simulink model "PlantaV4_6_prueba_contacto_4"  (R2021a)
settings: Solver=VariableStepAuto  StartTime=0.0  StopTime=60  MaxStep=1e-2  RelTol=1e-3
values from neighbouring files (symbols this model uses):
  ahmax = 0.75    [valoresPlanta_29_9_24.m]    (also in valoresPlanta_V3.m)
  alfahmax = ((2*ahmax)/(rhd))    (= 2)    [valoresPlanta_29_9_24.m]    (also in valoresPlanta_V3.m)
  alfatmax = atmax/rtd    (= 1.6)    [valoresPlanta_29_9_24.m]    (also in valoresPlanta_V3.m)
  atmax = 0.8    [valoresPlanta_29_9_24.m]    (also in valoresPlanta_V3.m)
  ax_max = 0.8    [valoresPlanta_29_9_24.m]    (also in valoresPlanta_v4.m)
  ay_max = 0.75    [valoresPlanta_29_9_24.m]    (also in valoresPlanta_v4.m)
  bcx = 1e6    (= 1000000)    [Valores_1.m]    (also in valoresPlanta.m; valoresPlanta_29_9_24.m; valoresPlanta_V3.m; valoresPlanta_v4.m)
  bcy = 1e7    (= 10000000)    [Valores_1.m]    (also in valoresPlanta.m; valoresPlanta_29_9_24.m; valoresPlanta_V3.m; valoresPlanta_v4.m)
  bh_eq = bhm*ih^2+bhd    (= 8720)    [Valores.m]    (also in Valores_1.m; valoresPlanta.m; valoresPlanta_29_9_24.m; valoresPlanta_V3.m)
  bhb = 1e8    (= 100000000)    [Valores.m]    (also in Valores_1.m; valoresPlanta.m; valoresPlanta_29_9_24.m; valoresPlanta_V3.m)
  bhEb = 2.2e9    (= 2200000000)    [Valores.m]    (also in Valores_1.m; valoresPlanta.m; valoresPlanta_29_9_24.m; valoresPlanta_V3.m)
  bt = 90.0    (= 90)    [Valores.m]    (also in Valores_1.m; valoresPlanta.m; valoresPlanta_29_9_24.m; valoresPlanta_V3.m)
  bt_eq = btd+(btm*(it^2))    (= 5401.8)    [valoresPlanta.m]    (also in valoresPlanta_29_9_24.m; valoresPlanta_V3.m; valoresPlanta_v4.m)
  btw = 3.0e3    (= 3000)    [Valores.m]    (also in Valores_1.m; valoresPlanta.m; valoresPlanta_29_9_24.m; valoresPlanta_V3.m)
  bwu = 150    [Valores.m]    (also in Valores_1.m; valoresPlanta.m; valoresPlanta_29_9_24.m; valoresPlanta_V3.m)
  estado_cont = [x_positions; hy_cont]    [perfilObsaculos.m]    (also in valoresPlanta_29_9_24.m = [x_positions; [hy_muelle hy_cont]])
  g = 9.80665    [Valores.m]    (also in Valores_1.m; valoresPlanta.m; valoresPlanta_29_9_24.m; valoresPlanta_V3.m)
  Hc = 0    [Valores.m]    (also in Valores_1.m = 2.5; valoresPlanta.m = 2.5; valoresPlanta_29_9_24.m = 2.5; valoresPlanta_V3.m = 2.5)
  hMax = 10    [Valores_1.m]    (also in valoresPlanta.m; valoresPlanta_V3.m; valoresPlanta_v4.m)
  hx_cont = 2.5    [perfilObsaculos.m]    (also in puntosTrayectoria.m; valoresPlanta_29_9_24.m)
  ih = 22    [Valores.m]    (also in Valores_1.m; valoresPlanta.m; valoresPlanta_29_9_24.m; valoresPlanta_V3.m)
  it = 30    [Valores.m]    (also in Valores_1.m; valoresPlanta.m; valoresPlanta_29_9_24.m; valoresPlanta_V3.m)
  Jh_eq = Jhm_hb*ih^2+Jhd_hEb    (= 18320)    [Valores.m]    (also in Valores_1.m; valoresPlanta.m; valoresPlanta_29_9_24.m; valoresPlanta_V3.m)
  Jt_eq = Jtd+(Jtm_tb*(it^2))    (= 7500)    [valoresPlanta.m]    (also in valoresPlanta_29_9_24.m; valoresPlanta_V3.m; valoresPlanta_v4.m)
  kcy = 1.8e9    (= 1800000000)    [Valores_1.m]    (also in valoresPlanta.m; valoresPlanta_29_9_24.m; valoresPlanta_V3.m; valoresPlanta_v4.m)
  KDh = Jeq2 * w_posh^3    (= -12245.4404091)    [Valores.m]    (also in Valores_1.m = Jeq2 * w_posh; valoresPlanta.m = Jeq2 * w_posh; valoresPlanta_29_9_24.m = Jh_eq * n * w_posh; valoresPlanta_V3.m = Jeq2 * w_posh)
  KDt = Meq2 * w_post^3    (= -4728.86946035)    [Valores.m]    (also in Valores_1.m = Meq2 * w_post; valoresPlanta.m = Meq2 * w_post; valoresPlanta_29_9_24.m = 10127; valoresPlanta_V3.m = Meq2 * w_post)
  KIh = Jeq2 * w_posh^2    (= 2572.66592082)    [Valores.m]    (also in Valores_1.m = Jeq2 * w_posh^3; valoresPlanta.m = Jeq2 * w_posh^3; valoresPlanta_29_9_24.m = Jh_eq * w_posh^3; valoresPlanta_V3.m = Jeq2 * w_posh^3)
  KIt = Meq2 * w_post^2    (= 1307.690244)    [Valores.m]    (also in Valores_1.m = Meq2 * w_post^3; valoresPlanta.m = Meq2 * w_post^3; valoresPlanta_29_9_24.m = 6809.6; valoresPlanta_V3.m = Meq2 * w_post^3)
  KPh = Jeq2 * w_posh    (= -540.495867769)    [Valores.m]    (also in Valores_1.m = Jeq2 * w_posh^2; valoresPlanta.m = Jeq2 * w_posh^2; valoresPlanta_29_9_24.m = Jh_eq * n * w_posh^2; valoresPlanta_V3.m = Jeq2 * w_posh^2)
  KPt = Meq2 * w_post    (= -361.62)    [Valores.m]    (also in Valores_1.m = Meq2 * w_post^2; valoresPlanta.m = Meq2 * w_post^2; valoresPlanta_29_9_24.m = 14123; valoresPlanta_V3.m = Meq2 * w_post^2)
  Ktw = 4.8e5    (= 480000)    [Valores.m]    (also in Valores_1.m; valoresPlanta.m; valoresPlanta_29_9_24.m; valoresPlanta_V3.m)
  kwu = 2.36e8    (= 236000000)    [Valores.m]    (also in Valores_1.m; valoresPlanta.m; valoresPlanta_29_9_24.m; valoresPlanta_V3.m)
  Mc_max = 5e4    (= 50000)    [Valores.m]    (also in Valores_1.m; valoresPlanta.m; valoresPlanta_29_9_24.m; valoresPlanta_V3.m)
  Mc_min = 2e3    (= 2000)    [Valores.m]    (also in Valores_1.m; valoresPlanta.m; valoresPlanta_29_9_24.m; valoresPlanta_V3.m)
  Meq = Mt+(it^2*Jtm_tb+Jtd)/rtd^2    (= 60000)    [Valores.m]    (also in Valores_1.m; valoresPlanta_29_9_24.m; valoresPlanta_v4.m)
  Ms = 1.5e4    (= 15000)    [Valores.m]    (also in Valores_1.m; valoresPlanta.m; valoresPlanta_29_9_24.m; valoresPlanta_V3.m)
  Mt = 30000    [Valores.m]    (also in Valores_1.m; valoresPlanta.m; valoresPlanta_29_9_24.m; valoresPlanta_V3.m)
  rhd = 0.75    [Valores.m]    (also in Valores_1.m; valoresPlanta.m; valoresPlanta_29_9_24.m; valoresPlanta_V3.m)
  rtd = 0.5    [Valores.m]    (also in Valores_1.m; valoresPlanta.m; valoresPlanta_29_9_24.m; valoresPlanta_V3.m)
  tau_hm = 1e-3    (= 0.001)    [valoresPlanta.m]    (also in valoresPlanta_29_9_24.m; valoresPlanta_V3.m; valoresPlanta_v4.m)
  tau_tm = 1e-3    (= 0.001)    [Valores.m]    (also in Valores_1.m; valoresPlanta.m; valoresPlanta_29_9_24.m; valoresPlanta_V3.m)
  Thb_Max = 5e4    (= 50000)    [Valores.m]    (also in Valores_1.m; valoresPlanta.m; valoresPlanta_29_9_24.m; valoresPlanta_V3.m)
  ThEb_Max = 1.1e6    (= 1100000)    [Valores.m]    (also in Valores_1.m; valoresPlanta.m; valoresPlanta_29_9_24.m; valoresPlanta_V3.m)
  Thm_Max = 2e4    (= 20000)    [Valores.m]    (also in Valores_1.m; valoresPlanta.m; valoresPlanta_29_9_24.m; valoresPlanta_V3.m)
  Ttb_Max = 5e3    (= 5000)    [Valores.m]    (also in Valores_1.m; valoresPlanta.m; valoresPlanta_29_9_24.m; valoresPlanta_V3.m)
  Ttm_Max = 3e3    (= 3000)    [Valores.m]    (also in Valores_1.m; valoresPlanta.m; valoresPlanta_29_9_24.m = 4000; valoresPlanta_V3.m)
  v_x_max = 4    [Valores_1.m]    (also in valoresPlanta.m; valoresPlanta_V3.m = 0.4; valoresPlanta_v4.m)
  vx_max = 4    [valoresPlanta_29_9_24.m]
  y0 = 2.5    [valoresPlanta_29_9_24.m]
  Yt0 = 45    [Valores.m]    (also in Valores_1.m; valoresPlanta.m; valoresPlanta_29_9_24.m; valoresPlanta_V3.m)
undefined symbols (not defined in the file or in its folder): sigbuilder_block, x0
libraries: vrlib x1, simulink_extras x1, cstblocks x1
(part 2 of 2)

== stateflow chart PlantaV4_6_prueba_contacto_4/Control Supervisor/Movimiento ==
  state estado_inicial [parallel] [commented out]
    entry:
    vYref = 0;
    vXref = 0;
    flag_carga = 1;
  state Movimiento [parallel] [commented out]
    entry:
    h_i = 0;
    h_seg = 0;
    %[h_i, h_seg] = calculaH1(v_x_max, dX, hMax, v_y_max,dh);
    %v_x_max = 4;
    during:
    v_y_max = calcVel(ml, g);
    %v_y_max = 2;
    h_i = 5;
    h_seg = 15;
    %[h_i, h_seg] = calculaH1(v_x_max, dX, hMax, v_y_max,dh);
    state Estado4 [commented out]
      entry:
      E = 4; %estado 4
      during:
      if (toDock==1)
      vYref = v_y_max; %suma
      vXref = v_x_max;  %cte desaceleracion hasta 0 (suma)
      else
      vYref = v_y_max; %suma
      vXref = 0.1;  %cte desaceleracion hasta 0
      end
    state Estado3 [commented out]
      entry:
      E = 3; %estado 3
      during:
      vYref = 0;
      if (toDock==1)
      vXref = -v_x_max;
      else
      vXref = v_x_max;
      end
    state Estado2 [commented out]
      entry:
      E = 2; %estado 2
      during:
      if (toDock==1)
      vYref = -v_y_max;
      vXref = -v_x_max;
      else
      vYref = v_y_max;
      vXref = v_x_max;
      end
    note: %ver de comparar con posicion objetivo
        | definir hmax (2 contenedores)
    state DescargaConteiner [commented out]
      entry:
      ml = Ms;
    state Estado5 [commented out]
      entry:
      E = 5; %estado 5
      during:
      if (toDock==1)
      vYref = vYref+0.5; %acelero
      vXref = 0;
      %ml = Ms;
      else
      vYref = vYref-0.5; %desacelero
      vXref = 0;
      end
    state Estado1 [commented out]
      entry:
      E = 1; %estado 1
      during:
      if (toDock==1)
      if (yl > 0)
      vYref = -v_y_max;
      end
      else
      vYref = v_y_max;
      if (yl < h_i)
      vYref = 0;
      end
      end
    state EstadoInicial [commented out]
      entry:
      entry:
      E = 0; %estado 0
      vYref = 0;
      vXref = 0;
      flag_carga = 0;
      ml = fcn(Mc_Max, Mc_Min);
    Estado3 -> Estado2 [commented out] : [xl<=dX && toDock==1 && yl >= h_seg]
    Estado3 -> Estado4 [commented out] : [xl>= posXref-7.5 && toDock==0]
    Estado2 -> Estado3 [commented out] : [xl>=dX && toDock==0 && yl >= h_seg]
    Estado4 -> Estado3 [commented out] : [xl<= posXref-7.5 && toDock==1]
    Estado4 -> Estado5 [commented out] : [yl==hMax && vXref<=0 && toDock==0]
    Estado5 -> Estado4 [commented out] : [yl==hMax && toDock==1]
    Estado2 -> Estado1 [commented out] : [yl<=h_i && toDock==1]
    Estado1 -> Estado2 [commented out] : [yl >= h_i && toDock==0]
    Estado5 -> DescargaConteiner [commented out] : [yl == posYref && toDock==0]
    DescargaConteiner -> EstadoInicial [commented out] : [Automatico == 1 && flag_carga == 1]
    (default) -> EstadoInicial [commented out]
    EstadoInicial -> Estado1 [commented out] : [Automatico == 1 && toDock==0]
    EstadoInicial -> Estado5 [commented out] : [Automatico == 1 && toDock==1]
    Estado1 -> EstadoInicial [commented out] : [Automatico == 1 && toDock==1]
  state Manual [parallel] [commented out]
  state estado_inicial1 [parallel] [commented out]
    entry:
    vYref = 0;
    vXref = 0;
    flag_carga = 1;
  state perfiles [parallel]
    entry:
    v_y_max = calcVel(ml, g);
    v_x_max = vx_max;
    during:
    h_i = pos(1,2);
    h_seg = pos(2,2);
    ds = pos(3,2) - pos(1,2);
    db = pos(4,2) - pos(6,2);
    y2 = ds - calcPos(ds, v_y_max, ahmax,0);
    y3 = db - calcPos(db, v_y_max, ahmax,0);
    %funcionaria para 1 ciclo, sino calcular x2 en carro
    %x2 = 10;
    dc = pos(5,1) - pos(2,1);
    x2 = dc - calcPos(dc, v_x_max, ax_max,0);
    vXref = 0;
    vYref = 0;
    settings: executionOrder=1
    state izaje1 [parallel]
      settings: executionOrder=2
      state inicial
        entry:
      state Izaje_subida
        state trayectoria
          entry:
          initialTime_y = currentTime;  %10
          % perfil de velocidad teniendo en cuenta el tiempo, no el espacio a alcanzar
          % totalTime: tiempo necesario para llegar al x final
          if (estado==1)
          PosFinal_y = pos(3,2)-pos(1,2);
          elseif (estado==6)
          PosFinal_y = pos2(3,2)-pos2(1,2);
          end
          %no se si se puede redefinir asi v_max
          [totalTime_y, v_y_max] = calcularTiempoTrapezoidal(PosFinal_y, v_y_max, ay_max);
          vYref = generateVelocityProfile(v_y_max, ay_max, currentTime, totalTime_y, initialTime_y);
          during:
          vYref = generateVelocityProfile(v_y_max, ay_max, currentTime, totalTime_y, initialTime_y);
        state detencion
          entry:
          vYref = 0;
          during:
          vYref = 0;
        perfiles.izaje1.Izaje_subida.trayectoria -> perfiles.izaje1.Izaje_subida.detencion : [estado==3 || estado == 8]
      state Izaje_bajada
        state trayectoria
          entry:
          initialTime_y = currentTime;  %10
          % perfil de velocidad teniendo en cuenta el tiempo, no el espacio a alcanzar
          % totalTime: tiempo necesario para llegar al x final
          if (estado == 4)
          PosFinal_y = abs(pos(6,2)-pos(4,2));
          elseif (estado == 9)
          PosFinal_y = abs(pos2(6,2)-pos2(4,2));
          end
          [totalTime_y, v_y_max] = calcularTiempoTrapezoidal(PosFinal_y, v_y_max, ay_max);
          vYref = - generateVelocityProfile(v_y_max, ay_max, currentTime, totalTime_y, initialTime_y);
          during:
          vYref = - generateVelocityProfile(v_y_max, ay_max, currentTime, totalTime_y, initialTime_y);
        state detencion
          entry:
          vYref = 0;
          during:
          vYref = 0;
        perfiles.izaje1.Izaje_bajada.trayectoria -> perfiles.izaje1.Izaje_bajada.detencion : [estado==6 || estado==11]
      perfiles.izaje1.inicial -> perfiles.izaje1.Izaje_subida.trayectoria : [estado == 1 || estado == 6]
      (default) -> perfiles.izaje1.inicial
      perfiles.izaje1.Izaje_subida.detencion -> perfiles.izaje1.Izaje_bajada.trayectoria : [estado == 4 || estado == 9]
    note: REVISAR
    note: para izaje es de 1 a 3 subida, de 4 a 6 bajada
        | CAMBIAR ESADOS PARA FRENAR
    state Carro_trapezoidal1 [parallel]
      settings: executionOrder=1
      state inicial
        entry:
        entry:
        vXref = 0;
        during:
        vXref = 0;
      state trayectoria
        entry:
        %v_x_max = vx_max;
        initialTime = currentTime;  %10
        % perfil de velocidad teniendo en cuenta el tiempo, no el espacio a alcanzar
        % totalTime: tiempo necesario para llegar al x final
        PosFinal = pos(5,1)-pos(2,1);
        [totalTime, v_x_max] = calcularTiempoTrapezoidal(PosFinal, v_x_max, ax_max);
        vXref = generateVelocityProfile(v_x_max, ax_max, currentTime, totalTime, initialTime);
        during:
        vXref = generateVelocityProfile(v_x_max, ax_max, currentTime, totalTime, initialTime);
      state trayectoria1 [commented out]
        entry:
        %v_x_max = vx_max;
        initialTime = currentTime;  %10
        % perfil de velocidad teniendo en cuenta el tiempo, no el espacio a alcanzar
        % totalTime: tiempo necesario para llegar al x final
        PosFinal = pos2(5,1)-pos2(2,1);
        [totalTime, v_x_max] = calcularTiempoTrapezoidal(PosFinal, v_x_max, ax_max);
        vXref = generateVelocityProfile(v_x_max, ax_max, currentTime, totalTime, initialTime);
        during:
        vXref = generateVelocityProfile(v_x_max, ax_max, currentTime, totalTime, initialTime);
      state detencion
        entry:
        vXref = 0;
        during:
        vXref = 0;
      state detencion1 [commented out]
        entry:
        vXref = 0;
        during:
        vXref = 0;
      (default) -> perfiles.Carro_trapezoidal1.inicial
      perfiles.Carro_trapezoidal1.inicial -> perfiles.Carro_trapezoidal1.trayectoria : [estado == 2]
      perfiles.Carro_trapezoidal1.trayectoria -> perfiles.Carro_trapezoidal1.detencion : [estado==5]
      perfiles.Carro_trapezoidal1.detencion -> trayectoria1 [commented out] : [estado==7]
      trayectoria1 -> detencion1 [commented out] : [estado==11]
    state Carro_trapezoidal [parallel] [commented out]
      state inicial [commented out]
      note: offset -20
      state Aceleracion [commented out]
        entry:
        %vYref = 0;
        aXref = 0;
        during:
        aXref = ax_max;
      state MRU [commented out]
        entry:
        aXref = 0;
        during:
        aXref = 0;
      state Desaceleracion [commented out]
        entry:
        aXref = 0;
        during:
        aXref = -ax_max;
      state Stop [commented out]
        during:
        aXref = 0;
      (default) -> perfiles.Carro_trapezoidal.inicial [commented out]
      perfiles.Carro_trapezoidal.inicial -> perfiles.Carro_trapezoidal.Aceleracion [commented out] : [estado==2]
      perfiles.Carro_trapezoidal.Desaceleracion -> perfiles.Carro_trapezoidal.Stop [commented out] : [vt<=0]
      perfiles.Carro_trapezoidal.MRU -> perfiles.Carro_trapezoidal.Desaceleracion [commented out] : [(xt)>=x2]
      perfiles.Carro_trapezoidal.Aceleracion -> perfiles.Carro_trapezoidal.MRU [commented out] : [vt>=v_x_max-0.455]
      perfiles.Carro_trapezoidal.Stop -> Carro_trapezoidal [commented out]
    state izaje [parallel] [commented out]
      state inicio [commented out]
      state Izaje_subida [commented out]
        note: calcular y 2
        state Aceleracion [commented out]
          entry:
          %vYref = 0;
          aYref = 0;
          during:
          aYref = ahmax;
        state MRU [commented out]
          entry:
          aYref = 0;
          during:
          aYref = 0;
        state Desaceleracion [commented out]
          entry:
          aYref = 0;
          during:
          aYref = -ahmax;
        state Stop [commented out]
          during:
          aYref = 0;
        (default) -> perfiles.izaje.Izaje_subida.Aceleracion [commented out]
        perfiles.izaje.Izaje_subida.Desaceleracion -> perfiles.izaje.Izaje_subida.Stop [commented out] : [vh<=0]
        perfiles.izaje.Izaje_subida.MRU -> perfiles.izaje.Izaje_subida.Desaceleracion [commented out] : [yl>=y2]
        perfiles.izaje.Izaje_subida.Aceleracion -> perfiles.izaje.Izaje_subida.MRU [commented out] : [vh>=v_y_max]
      state Izaje_bajada [commented out]
        note: REVISAR
        state Aceleracion [commented out]
          entry:
          %vYref = 0;
          aYref = 0;
          during:
          aYref = -ahmax;
        state MRU [commented out]
          entry:
          aYref = 0;
          during:
          aYref = 0;
        state Desaceleracion [commented out]
          entry:
          aYref = 0;
          during:
          aYref = ahmax;
        state Stop [commented out]
          during:
          aYref = 0;
        (default) -> perfiles.izaje.Izaje_bajada.Aceleracion [commented out]
        perfiles.izaje.Izaje_bajada.Desaceleracion -> perfiles.izaje.Izaje_bajada.Stop [commented out] : [vh>=0]
        perfiles.izaje.Izaje_bajada.MRU -> perfiles.izaje.Izaje_bajada.Desaceleracion [commented out] : [abs(pos(4,2)-yl)>=abs(y3)]
        perfiles.izaje.Izaje_bajada.Aceleracion -> perfiles.izaje.Izaje_bajada.MRU [commented out] : [abs(vh)>=v_y_max]
      (default) -> inicio [commented out]
      inicio -> perfiles.izaje.Izaje_subida [commented out] : [estado == 1]
      perfiles.izaje.Izaje_subida.Stop -> perfiles.izaje.Izaje_bajada [commented out] : [estado == 4]
  state estados [parallel]
    entry:
    pos = calcularTrayectoria2_prueba(vx_max, v_y_max, ax_max, Hc, hx_cont, [30.5,30], [-20,2.5], 0, estado_cont)
    pos2 = calcularTrayectoria2_prueba(vx_max, v_y_max, ax_max, Hc, hx_cont, [-10.5,30], [30.5,30], 0, estado_cont)
    settings: executionOrder=2
    note: (abs(yl-pos(3,2))<0.2
    state e3
      entry:
      estado = 3;
    state e4
      entry:
      estado = 4;
    state e8
      entry:
      estado = 8;
    state e9
      entry:
      estado = 9;
    note: -20 arrancamos de -20. corregir
    state e2
      entry:
      estado = 2;
    state e5
      entry:
      estado = 5;
    state e7
      entry:
      estado = 7;
    state e10
      entry:
      estado = 10;
    state e1
      entry:
      estado = 1;
    state e6
      entry:
      estado = 6;
    state e11
      entry:
      estado = 11;
    note: agregar esado inicial
        | conrolar la velocidad para que no se pase del maximo
    e4 -> e5 : [((xt) >=pos(5,1)) && (yl >=pos(5,2))]
    e9 -> e10 : [((xt) >=pos2(5,1)) && (yl >=pos2(5,2))]
    e8 -> e9 : [(ciclo == 1) && ((xt) >=pos2(4,1))]
    e2 -> e3 : [(((xl)>pos(3,1))) && (yl>pos(3,2)-0.2)]
    e3 -> e4 : [((xt) >=pos(4,1))]
    e7 -> e8 : [(ciclo == 1) && (((xl)>pos2(3,1))) && (yl>pos2(3,2)-0.2)]
    e1 -> e2 : [(yl >=pos(2,2))]
    e5 -> e6 : [(abs((xl)-pos(6,1))<=0.2) && (yl >=pos(6,2))]
    e6 -> e7 : [(ciclo == 1) &&  (yl >=pos2(2,2))]
    e10 -> e11 : [(abs((xl)-pos2(6,1))<=0.2) && (yl >=pos2(6,2))]
    (default) -> e1
  (default) -> estado_inicial [commented out]
  estado_inicial -> Manual [commented out] : [Automatico == 0]
  estado_inicial -> Movimiento [commented out] : [Automatico == 1]
  Movimiento -> Manual [commented out] : [Automatico == 0]
  Manual -> Movimiento [commented out] : [Automatico == 1]
  (default) -> estado_inicial1 [commented out]
  estado_inicial1 -> ? [commented out] : [Automatico == 1]
  data: Ml function_input; vMaxY function_output; G function_input; DIS function_input; dx function_output; V function_input; A function_input; x0 function_input; v_max function_input; a_max function_input; current_time function_input; total_time function_input; next_velocity function_output; initial_time function_input; posicion_final function_input; velocidad_maxima function_input; aceleracion_maxima function_input; tiempo function_output; velocidad_corregida function_output; VX_MAX function_input; VY_MAX function_input; AX_MAX function_input; dy function_input; anchoCont function_input; pos_f function_input; pos_i function_input; to_where function_input; estado_cont function_input; pos function_output; Automatico input =1; v_y_max local; toDock input; xl input; yl input; v_x_max local; vh input; vt input; hMax parameter; h_i local; h_seg local; g parameter; Ms parameter; E local; flag_carga local; ml input; xt input; pos local; estado local; db local; ds local; y2 local; y3 local; x2 local; ahmax parameter; ax_max parameter; dc local; currentTime input; vXref output; PosFinal local; initialTime local; totalTime local; PosFinal_y local; initialTime_y local; totalTime_y local; vYref output; ay_max parameter; vx_max parameter; ciclo input; Hc parameter; estado_cont parameter; hx_cont parameter; pos2 local
  function vMaxY = calcVel(Ml, G):
    | function vMaxY = calcVel(Ml, G)
    | %  vMaxY = 956.15e3/((Ml)*G);
    | % Valor de potencia constante a cumplir
    | Pconst = 65000*9.80665*1.5;
    | vMaxY = 1.5;
    | 
    | % Determinacion de velocidad del izaje segun masa de carga
    | if (Ml <= 32500)
    |     vMaxY = 3;
    | 
    | elseif (Ml <65000)
    |     vMaxY = Pconst / (Ml * g);
    | elseif (Ml >= 65000)
    |     vMaxY = 1.5;
    | end
    | 
    | end
  function dx = calcPos(DIS, V, A, x0):
    | function dx = calcPos(DIS, V, A, x0)
    | %12m es la dis minima para desarrollar max velocidad a Amax 
    | % if DIS<12
    | %     dx = DIS - DIS/3;    %3er tercio
    | % else
    | %     dx = v^2/(2*a);    %para izaje 
    | % end
    | dx = x0 + V^2/(2*A);    %para izaje
    | %si DIS < 2*dx ahi divido en 3
    | end
  function next_velocity = generateVelocityProfile(v_max, a_max, current_time, total_time, initial_time):
    | function next_velocity = generateVelocityProfile(v_max, a_max, current_time, total_time, initial_time)
    |     % Parámetros de tiempo
    |     t_acceleration = v_max / a_max;  % Tiempo de aceleración para alcanzar v_max
    |     t_constant = (total_time - 2 * t_acceleration);  % Tiempo en velocidad constante
    |     
    |     % Ajuste el tiempo actual para tener en cuenta el tiempo inicial
    |     current_time_adjusted = current_time - initial_time;
    |     if current_time_adjusted <= 0
    |         next_velocity = 0;
    |     elseif current_time_adjusted <= t_acceleration
    |         next_velocity = a_max * current_time_adjusted;
    |     elseif current_time_adjusted > t_acceleration && current_time_adjusted < (total_time - t_acceleration)
    |         next_velocity = v_max;
    |     else
    |         time_in_deceleration = total_time - current_time_adjusted;
    |         if time_in_deceleration < 0
    |             next_velocity = 0;
    |         else
    |             next_velocity = v_max - a_max * (current_time_adjusted - t_acceleration - t_constant);
    |         end
    |     end
    | end
    | 
    | % function next_velocity = generateVelocityProfile(v_max, a_max, current_time, total_time)
    | %     % Parámetros de tiempo
    | %     t_acceleration = v_max / a_max;  % Tiempo de aceleración para alcanzar v_max
    | %     t_constant = (total_time - 2 * t_acceleration);  % Tiempo en velocidad constante
    | %     if current_time <= t_acceleration
    | %         next_velocity = a_max * current_time;
    | %     elseif current_time > t_acceleration && current_time < (total_time - t_acceleration)
    | %         next_velocity = v_max;
    | %     else
    | %         time_in_deceleration = total_time - current_time;
    | %         if time_in_deceleration < 0
    | %             next_velocity = 0;
    | %         else
    | %             next_velocity = v_max - a_max * (current_time - t_acceleration - t_constant);
    | %             %tiempo de desaceleracion: tiempo total - tiempo total acel - tiempo cte 
    | %         end
    | %     end
    | % end
  function [tiempo, velocidad_corregida] = calcularTiempoTrapezoidal(posicion_final, velocidad_maxima, aceleracion_maxima):
    | function [tiempo, velocidad_corregida] = calcularTiempoTrapezoidal(posicion_final, velocidad_maxima, aceleracion_maxima)
    |     % Calcula el tiempo necesario para una trayectoria trapezoidal
    |     
    |     % Verifica si la velocidad máxima es alcanzable con la aceleración máxima
    |     tiempo_aceleracion = velocidad_maxima / aceleracion_maxima;
    |     distancia_aceleracion = 0.5 * velocidad_maxima * tiempo_aceleracion;
    |     
    |     % Calcula la distancia total a recorrer
    |     distancia_total = abs(posicion_final);
    |     
    |     if distancia_total <= 2 * distancia_aceleracion
    |         % No se alcanza la velocidad máxima, la aceleración es limitante
    |         % Calcula el tiempo necesario
    | %         tiempo = 2 * sqrt((distancia_total/2) / aceleracion_maxima);
    |         % d = vo * t + 1/2 * a * t^2
    | %         tiempo = sqrt(2 * distancia_total / aceleracion_maxima);
    |         % Calcula la velocidad corregida
    |         % vf = vo + a * t
    | %         velocidad_corregida = sqrt(2 * aceleracion_maxima * distancia_total);
    | %         velocidad_corregida = aceleracion_maxima * tiempo/2;
    |         d = distancia_total/3;    %perfil trapezoidal -> equidistante
    |         t1 = sqrt((2 * d)/aceleracion_maxima)
    |         % vf = vo + a * t
    |         velocidad_corregida = aceleracion_maxima * t1;
    |         t2 = d / velocidad_corregida;
    |         
    |         tiempo = (2 * t1) + t2;
    |         
    |     else
    |         % Se alcanza la velocidad máxima
    |         tiempo_desaceleracion = velocidad_maxima / aceleracion_maxima;
    |         tiempo = tiempo_aceleracion + (distancia_total - 2 * distancia_aceleracion) / velocidad_maxima + tiempo_desaceleracion;
    |         velocidad_corregida = velocidad_maxima;
    |     end
    | end
    | 
    | 
    | 
    | % function [tiempo, VX_MAX] = calcularTiempoTrapezoidal(posicion_final, velocidad_maxima, aceleracion_maxima)
    | % % si la distancia es demasiado pequeña para poder desarrollar la velocidad,
    | % % reducir la velocidad maxima 
    | % % La salida debe ser la velocidad maxima modificada, o la velocidad maxima
    | % 
    | % % Calcula el tiempo necesario para una trayectoria trapezoidal
    | %     
    | %     % Verifica si la velocidad máxima es alcanzable con la aceleración máxima
    | %     tiempo_aceleracion = velocidad_maxima / aceleracion_maxima;
    | %     distancia_aceleracion = 0.5 * velocidad_maxima * tiempo_aceleracion;
    | %     
    | %     % Calcula el tiempo necesario para desacelerar desde la velocidad máxima
    | %     tiempo_desaceleracion = velocidad_maxima / aceleracion_maxima;
    | %     
    | %     % Calcula la distancia total a recorrer
    | %     distancia_total = abs(posicion_final);
    | %     
    | %     if distancia_total <= 2 * distancia_aceleracion
    | %         % No se alcanza la velocidad máxima, la aceleración es limitante
    | %         
    | %         % Se corrige la velocidad, se mantiene la aceleracion maxima
    | %         VX_MAX = sqrt(2 * aceleracion_maxima * distancia_total/2);
    | %         
    | %         % Es correcto?? 
    | %         tiempo = 2 * sqrt((distancia_total / 2) / aceleracion_maxima);
    | %     else
    | %         % Se alcanza la velocidad máxima
    | %         tiempo = tiempo_aceleracion + (distancia_total - 2 * distancia_aceleracion) / velocidad_maxima + tiempo_desaceleracion;
    | %         VX_MAX = velocidad_maxima;
    | %     end
    | % end
  function pos= calcularTrayectoria2_prueba(VX_MAX, VY_MAX, AX_MAX, dy, anchoCont, pos_f, pos_i, to_where, estado_cont):
    | function pos= calcularTrayectoria2_prueba(VX_MAX, VY_MAX, AX_MAX, dy, anchoCont, pos_f, pos_i, to_where, estado_cont)
    |   ysb = 15;
    |     xi = pos_i(1);
    |     yi = pos_i(2);
    |     xf = pos_f(1);
    |     yf = pos_f(2);
    | 
    |     %pos_i y pos_f son vectores (x,y)
    |     theta = atan2(VY_MAX,VX_MAX);   %angulo para alcanzar ambas velocidades máximas
    |     fprintf('Distancia dx para alcanzar v. maximas');
    |     dx = (VX_MAX^2)/(2 * AX_MAX);
    | 
    |     if (2 * dx <= (xf-xi))
    |         fprintf('[index, hmax] para 2 * dx <= (xf-xi)\n');
    |         [hmax, index] = calcularIndice(xi, xf, anchoCont, to_where, estado_cont);
    |         disp(hmax);
    |         hp = tan(theta) * dx;
    |     else 
    |         fprintf('[index, hmax] para 2 * dx > (xf-xi)\n');
    |         [hmax, index] = calcularIndice(xi, xf, anchoCont, to_where, estado_cont);
    |         disp(hmax);
    |         VX_MAX = sqrt(2 * AX_MAX * abs((xf-xi)/2));
    |         theta = atan2(VY_MAX,VX_MAX);
    |         dx = (xf-xi)/2;
    |         hp = tan(theta) * dx;
    | %     else (dx > (xf-xi)/2)
    | %         [index, hmax] = calcularIndice(xl, anchoCont, to_where, estado_cont)
    | %         VX_MAX = sqrt(2 * AX_MAX * (xf-xi)/2);
    | %         theta = atan2(VY_MAX/VX_MAX);
    | %         dx = (xf-xi)/2
    | %         hp = tan(theta) * dx;
    | %     else
    | %         [index, hmax] = calcularIndice(xl, anchoCont, to_where, estado_cont)    
    | %         hp = tan(theta) * dx;
    |     end
    | 
    |      
    |     % si hmax es negativo, lo hago ser 15
    |     if (hmax < 0)
    |         hmax = ysb;
    |         % cambiar la altura
    |     elseif (hmax <= yf)
    |         hmax = yf + dy;
    |     end
    |         
    |     hseg = hmax + 2 * dy;  %altura de seguridad
    |     %hseg debe ser < 40:
    |     if ((hmax + 2*dy) >= 40)
    |         h_seg = 40;
    |     else
    |         h_seg = hmax + 2*dy;
    |     end
    | 
    |     p0 = [xi, yi];
    |     p1 = [xi, hmax];    %es muy jugado, puede chocar si la altura max es indice 1
    |     p2 = [(xi+dx), (hseg)];
    |     p3 = [(xf-dx), (hseg)];
    |     p4 = [xf, hmax];    %debe ser mayor a yf
    |     p5 = [xf, yf];
    |     pos = [p0; p1; p2; p3; p4; p5];
    | end
    |     
    |     
    |  
    | function [hmax, index_max] = calcularIndice(xi, xf, anchoCont, ~, estado_cont)
    |     % Calcular el índice del valor más alto
    |     % Debe arrancar desde el inicio (-30), no desde el muelle
    |     % indice negativo: solucionado
    |     % 
    |     fprintf('index\n')
    |     index = floor((xi) / anchoCont); % extremo: -11 --> 1
    |     % hacer: floor((xi) / anchoCont) + 1 + 12 (para arrancar en 1.25) 
    |     index = index + 12;
    |     
    |     fprintf('index_obj\n')
    |     index_obj = floor((xf) / anchoCont);
    |     index_obj = index_obj + 12;
    |     
    |     % Verificar la dirección --> usar posiciones en coordenadas
    |     if (index_obj > index)
    |         fprintf('index_obj > index\n')
    |         % Calcular la altura máxima para índices menores al calculado
    |         [hmax, index_max] = max(estado_cont(2,index:index_obj)); %posible error: indice de subelemento
    |         index_max = index_max + index -1;
    |     elseif (index_obj < index)
    |         fprintf('index_obj < index\n')
    |         %comparar posicion objetivo con la inicial
    |         [hmax, index_max] = max(estado_cont(2,index_obj:index));
    |         index_max = index_max + index_obj - 1;
    |     else
    |         fprintf('No deberia activarse\n')
    |         % Otra opción no especificada
    |         hmax = 0;
    |         index_max = 0;
    |         fprintf('Dirección no válida');
    |     end
    | 
    | end
    | 
    | 
    | 
    | % % Verificar la dirección --> usar posiciones en coordenadas
    | % if (to_where == 0)
    | %     % Calcular la altura máxima para índices menores al calculado
    | %     hmax = max(estado_cont(1:index));
    | % elseif (to_where == 1)
    | %     % Calcular la altura máxima para índices mayores/menores al calculado
    | %     %comparar posicion objetivo con la inicial
    | %     hmax = estado_cont(index);
    | % elseif (to_where == 2)
    | %     % Calcular la altura máxima para índices mayores al calculado
    | %     hmax = max(estado_cont(index:end));
    | % else
    | %     % Otra opción no especificada
    | %     error('Dirección no válida');
    | % end

== matlab function PlantaV4_6_prueba_contacto_4/Control Supervisor/fcn ==
  data: Mc_Max input; Mcx output; Mc_Min input; flag_carga input
function Mcx = fcn(Mc_Max, Mc_Min, flag_carga)
%Agregar: sobrecarga
if (flag_carga == 1)
    Mcx = Mc_Min + (Mc_Max - Mc_Min)*rand(1);
    %ml = Mc_Max + 0.01 * randi([1,15],1) * Mc_Max;
else
    Mcx = 0;
end
end
